simulink model "controlPosicion_OK"  (R2019b)
settings: Solver=VariableStepAuto  StartTime=0.0  StopTime=10  FixedStep=0.005  RelTol=1e-3
values from neighbouring files (symbols this model uses):
  kp = 100    [Calculo_Tau_RR.m]
  kv = 2*sqrt(kp)    [Calculo_Tau_RR.m]
libraries: roblocks x17
settings Model: Creator=Marcelo  LastModifiedBy=rochi
settings DebuggingCC: ArithmeticOperatorsInVariantConditions=warning
settings SFSimCC: CustomCodeUndefinedFunction=UseInterfaceOnly

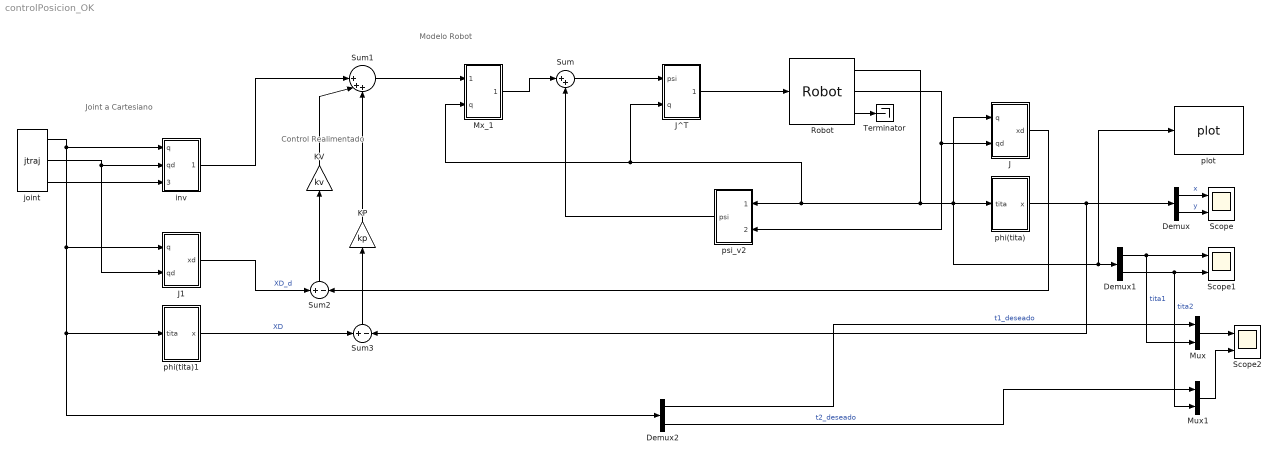
== system controlPosicion_OK ==
  note: Control Realimentado
  note: Modelo Robot
  note: Joint a Cartesiano
  Demux : Demux  Outputs=2
  Demux1 : Demux  Outputs=2
  Demux2 : Demux  Outputs=2
  J : Subsystem
  J1 : Subsystem
  J^T : Subsystem
  KP : Gain  Gain=kp
  KV : Gain  Gain=kv
  Mux : Mux  Inputs=2
  Mux1 : Mux  Inputs=2
  Mx_1 : Subsystem
  Robot : roblocks/Arm/Robot  robot=Robot  q0=[0 -pi/2]
  Scope : Scope  NumInputPorts=2
  Scope1 : Scope  NumInputPorts=2
  Scope2 : Scope  NumInputPorts=2
  Sum : Sum  Inputs=|++
  Sum1 : Sum  Inputs=||+++
  Sum2 : Sum  Inputs=+|-
  Sum3 : Sum  Inputs=+|-
  Terminator : Terminator
  inv : Subsystem
  joint : roblocks/Toolbox/jtraj  q0=[0 -pi/2]  qf=[pi/2 -pi/2]  tmax=10  ts=0.02
  phi(tita) : Subsystem
  phi(tita)1 : Subsystem
  plot : roblocks/Arm/plot  robot=Robot  fps=5  holdplot=on
  psi_v2 : Subsystem
  wires:
  Robot/2 -> psi_v2/2(tita_d), J/2(qd)
  KP/1 -> Sum1/3
  KV/1 -> Sum1/2
  Sum3/1 -> KP/1
  Sum2/1 -> KV/1
  phi(tita)/1(x) -> Sum3/2, Demux/1
  Demux/1 -> Scope/1  "x"
  Demux/2 -> Scope/2  "y"
  Demux1/2 -> Mux1/2, Scope1/2  "tita2"
  Demux1/1 -> Mux/2, Scope1/1  "tita1"
  J^T/1(tau) -> Robot/1
  J/1(xd) -> Sum2/2
  Robot/1 -> J/1(q), phi(tita)/1(tita), plot/1, Demux1/1, psi_v2/1(tita), Mx_1/2(q), J^T/2(q)
  psi_v2/1(psi) -> Sum/2
  Mx_1/1(psi_o) -> Sum/1
  Sum1/1 -> Mx_1/1(x_dd)
  Mux/1 -> Scope2/1
  Mux1/1 -> Scope2/2
  Demux2/1 -> Mux/1  "t1_deseado"
  Demux2/2 -> Mux1/1  "t2_deseado"
  Sum/1 -> J^T/1(psi)
  J1/1(xd) -> Sum2/1  "XD_d"
  phi(tita)1/1(x) -> Sum3/1  "XD"
  joint/1 -> inv/1(q), J1/1(q), Demux2/1, phi(tita)1/1(tita)
  joint/2 -> inv/2(qd), J1/2(qd)
  inv/1(xdd) -> Sum1/1
  joint/3 -> inv/3(qdd)
  Robot/3 -> Terminator/1

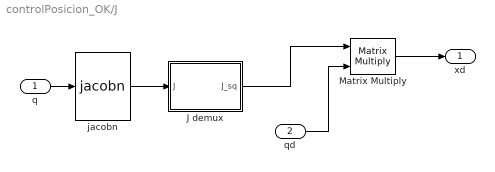
== system controlPosicion_OK/J ==
  q : Inport
  qd : Inport  Port=2
  J demux : MATLAB Function  TreatAsAtomicUnit=on
  Matrix Multiply : Product  Multiplication=Matrix(*)
  jacobn : roblocks/Arm/jacobn  robot=Robot
  xd : Outport
  wires:
  jacobn/1 -> J demux/1(J)
  qd/1 -> Matrix Multiply/2
  q/1 -> jacobn/1
  J demux/1(J_sq) -> Matrix Multiply/1
  Matrix Multiply/1 -> xd/1

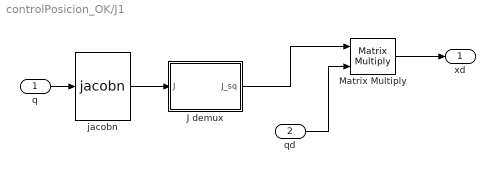
== system controlPosicion_OK/J1 ==
  q : Inport
  qd : Inport  Port=2
  J demux : MATLAB Function  TreatAsAtomicUnit=on
  Matrix Multiply : Product  Multiplication=Matrix(*)
  jacobn : roblocks/Arm/jacobn  robot=Robot
  xd : Outport
  wires:
  jacobn/1 -> J demux/1(J)
  qd/1 -> Matrix Multiply/2
  q/1 -> jacobn/1
  J demux/1(J_sq) -> Matrix Multiply/1
  Matrix Multiply/1 -> xd/1

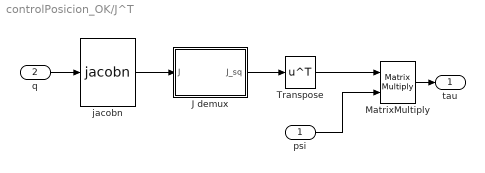
== system controlPosicion_OK/J^T ==
  psi : Inport
  q : Inport  Port=2
  J demux : MATLAB Function  TreatAsAtomicUnit=on
  MatrixMultiply : Product  Multiplication=Matrix(*)
  Transpose : Math  Operator=transpose  SaturateOnIntegerOverflow=on
  jacobn : roblocks/Arm/jacobn  robot=Robot
  tau : Outport
  wires:
  MatrixMultiply/1 -> tau/1
  q/1 -> jacobn/1
  jacobn/1 -> J demux/1(J)
  J demux/1(J_sq) -> Transpose/1
  Transpose/1 -> MatrixMultiply/1
  psi/1 -> MatrixMultiply/2

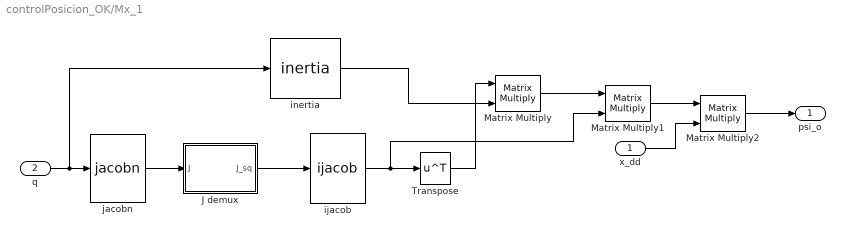
== system controlPosicion_OK/Mx_1 ==
  x_dd : Inport
  q : Inport  Port=2
  J demux : MATLAB Function  TreatAsAtomicUnit=on
  Matrix Multiply : Product  Multiplication=Matrix(*)
  Matrix Multiply1 : Product  Multiplication=Matrix(*)
  Matrix Multiply2 : Product  Multiplication=Matrix(*)
  Transpose : Math  Operator=transpose  SaturateOnIntegerOverflow=on
  ijacob : roblocks/Arm/ijacob
  inertia : roblocks/Arm/inertia  robot=Robot
  jacobn : roblocks/Arm/jacobn  robot=Robot
  psi_o : Outport
  wires:
  ijacob/1 -> Matrix Multiply1/2, Transpose/1
  Matrix Multiply1/1 -> Matrix Multiply2/1
  q/1 -> inertia/1, jacobn/1
  Transpose/1 -> Matrix Multiply/1
  J demux/1(J_sq) -> ijacob/1
  Matrix Multiply/1 -> Matrix Multiply1/1
  Matrix Multiply2/1 -> psi_o/1
  jacobn/1 -> J demux/1(J)
  x_dd/1 -> Matrix Multiply2/2
  inertia/1 -> Matrix Multiply/2

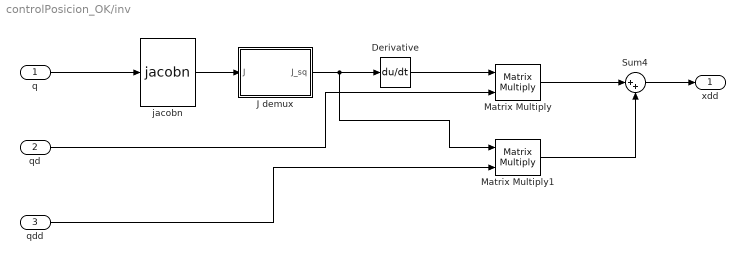
== system controlPosicion_OK/inv ==
  q : Inport
  qd : Inport  Port=2
  qdd : Inport  Port=3
  Derivative : Derivative
  J demux : MATLAB Function  TreatAsAtomicUnit=on
  Matrix Multiply : Product  Multiplication=Matrix(*)
  Matrix Multiply1 : Product  Multiplication=Matrix(*)
  Sum4 : Sum  Inputs=|++
  jacobn : roblocks/Arm/jacobn  robot=Robot
  xdd : Outport
  wires:
  Matrix Multiply/1 -> Sum4/1
  q/1 -> jacobn/1
  J demux/1(J_sq) -> Matrix Multiply1/1, Derivative/1
  Matrix Multiply1/1 -> Sum4/2
  qd/1 -> Matrix Multiply/2
  Sum4/1 -> xdd/1
  qdd/1 -> Matrix Multiply1/2
  jacobn/1 -> J demux/1(J)
  Derivative/1 -> Matrix Multiply/1

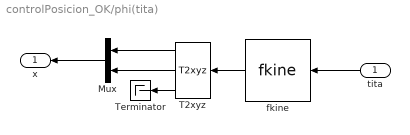
== system controlPosicion_OK/phi(tita) ==
  tita : Inport
  Mux : Mux  Inputs=2
  T2xyz : roblocks/Toolbox/T2xyz
  Terminator : Terminator
  fkine : roblocks/Arm/fkine  robot=Robot
  x : Outport
  wires:
  T2xyz/2 -> Mux/2
  Mux/1 -> x/1
  fkine/1 -> T2xyz/1
  tita/1 -> fkine/1
  T2xyz/1 -> Mux/1
  T2xyz/3 -> Terminator/1

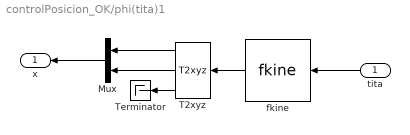
== system controlPosicion_OK/phi(tita)1 ==
  tita : Inport
  Mux : Mux  Inputs=2
  T2xyz : roblocks/Toolbox/T2xyz
  Terminator : Terminator
  fkine : roblocks/Arm/fkine  robot=Robot
  x : Outport
  wires:
  T2xyz/2 -> Mux/2
  Mux/1 -> x/1
  fkine/1 -> T2xyz/1
  tita/1 -> fkine/1
  T2xyz/1 -> Mux/1
  T2xyz/3 -> Terminator/1

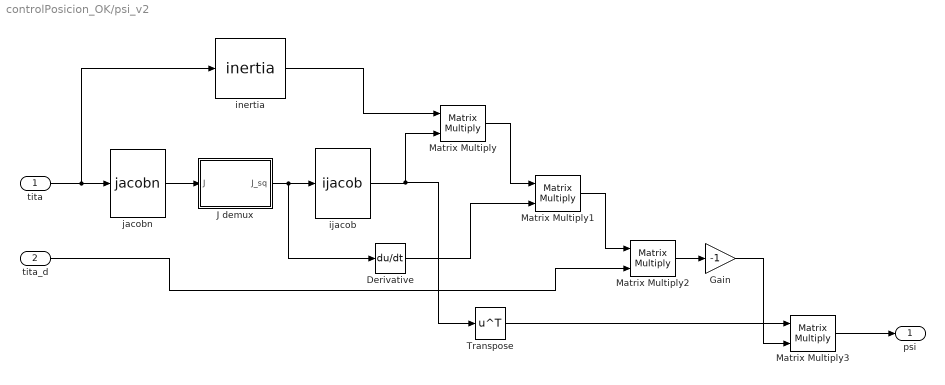
== system controlPosicion_OK/psi_v2 ==
  tita : Inport
  tita_d : Inport  Port=2
  Derivative : Derivative
  Gain : Gain  Gain=-1
  J demux : MATLAB Function  TreatAsAtomicUnit=on
  Matrix Multiply{,1..3} (4 alike) : Product  Multiplication=Matrix(*)
  Transpose : Math  Operator=transpose  SaturateOnIntegerOverflow=on
  ijacob : roblocks/Arm/ijacob
  inertia : roblocks/Arm/inertia  robot=Robot
  jacobn : roblocks/Arm/jacobn  robot=Robot
  psi : Outport
  wires:
  inertia/1 -> Matrix Multiply/1
  Matrix Multiply/1 -> Matrix Multiply1/1
  tita/1 -> inertia/1, jacobn/1
  tita_d/1 -> Matrix Multiply2/2
  ijacob/1 -> Transpose/1, Matrix Multiply/2
  J demux/1(J_sq) -> Derivative/1, ijacob/1
  Derivative/1 -> Matrix Multiply1/2
  jacobn/1 -> J demux/1(J)
  Matrix Multiply1/1 -> Matrix Multiply2/1
  Matrix Multiply3/1 -> psi/1
  Transpose/1 -> Matrix Multiply3/1
  Matrix Multiply2/1 -> Gain/1
  Gain/1 -> Matrix Multiply3/2

== matlab function controlPosicion_OK/J^T/J demux ==
  data: J input; J_sq output
function J_sq = fcn(J)

J_sq = [J(1,1) J(1,2);J(2,1) J(2,2)];

== matlab function controlPosicion_OK/J1/J demux ==
  data: J input; J_sq output
function J_sq = fcn(J)

J_sq = [J(1,1) J(1,2);J(2,1) J(2,2)];

== matlab function controlPosicion_OK/Mx_1/J demux ==
  data: J input; J_sq output
function J_sq = fcn(J)

J_sq = [J(1,1) J(1,2);J(2,1) J(2,2)];

== matlab function controlPosicion_OK/J/J demux ==
  data: J input; J_sq output
function J_sq = fcn(J)

J_sq = [J(1,1) J(1,2);J(2,1) J(2,2)];

== matlab function controlPosicion_OK/psi_v2/J demux ==
  data: J input; J_sq output
function J_sq = fcn(J)

J_sq = [J(1,1) J(1,2);J(2,1) J(2,2)];

== matlab function controlPosicion_OK/inv/J demux ==
  data: J input; J_sq output
function J_sq = fcn(J)

J_sq = [J(1,1) J(1,2);J(2,1) J(2,2)];
